simulink model "test"  (R2025b)
settings: Solver=ode8  StartTime=0.0  StopTime=4  RelTol=1e-3
libraries: simulink x4, dspfdesign x3, Monika x2
settings Model: VariantFading=off  Creator=maxim  LastModifiedBy=maxim

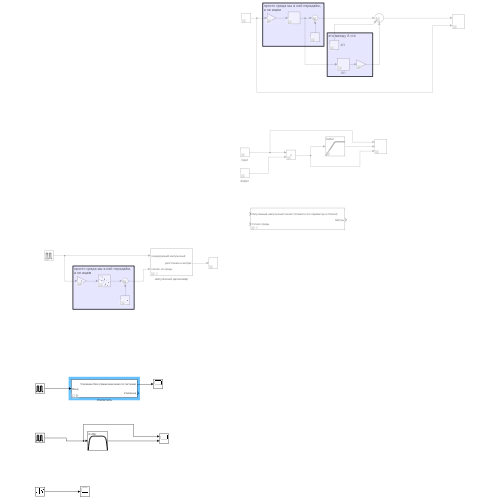
[thumbnail: Simulink's stored preview of the top-level diagram]
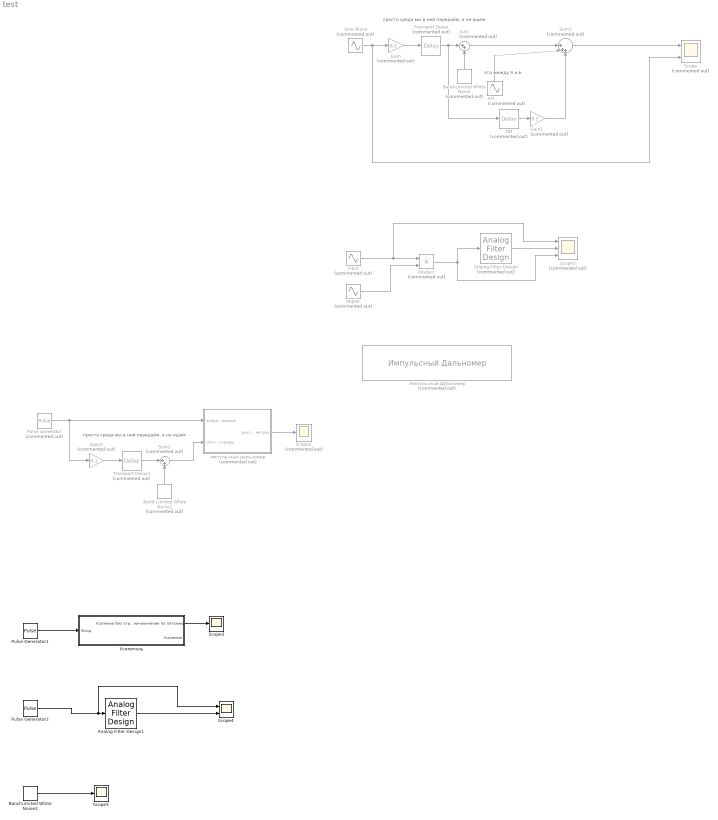
== system test ==
  note: это между А и Ь
  note: просто среда мы в ней передаём,
      | а не ищем
  note: просто среда мы в ней передаём,
      | а не ищем
  Analog Filter Design : dspfdesign/Analog Filter Design  Commented=on  method=Butterworth  filttype=Highpass  N=8  Wlo=20+8  Whi=80  Rp=2  Rs=40
  Analog Filter Design1 : dspfdesign/Analog Filter Design  method=Butterworth  filttype=Bandpass  N=2  Wlo=0.001  Whi=10  Rp=2  Rs=40
  Band-Limited White Noise : simulink/Sources/Band-Limited White Noise  Commented=on  Cov=[0.001]  Ts=0.001  seed=[23341]
  Band-Limited White Noise1 : simulink/Sources/Band-Limited White Noise  Commented=on  Cov=[0.001]  Ts=0.001  seed=[23341]
  Band-Limited White Noise2 : simulink/Sources/Band-Limited White Noise  Cov=0  Ts=0.00001  seed=[23341]
  Gain : Gain  Commented=on  Gain=0.1
  Gain1 : Gain  Commented=on  Gain=0.2
  Gain2 : Gain  Commented=on  Gain=0.1
  Product : Product  Commented=on
  Pulse Generator : DiscretePulseGenerator  Commented=on  PulseType=Time based  Period=1
  Pulse Generator1 : DiscretePulseGenerator  PulseType=Time based  Period=1  PulseWidth=10
  Pulse Generator2 : DiscretePulseGenerator  PulseType=Time based  Period=1  PulseWidth=10
  Scope : Scope  Commented=on  NumInputPorts=2
      settings: ActiveDisplayYMinimum=-12.499999674694067  ActiveDisplayYMaximum=12.499999961980945
  Scope1 : Scope  Commented=on  NumInputPorts=3
      settings: ActiveDisplayYMinimum=-1.2499999762577283  ActiveDisplayYMaximum=1.2499999284292547
  Scope2 : Scope  Commented=on
      settings: ActiveDisplayYMinimum=-206249.99999999994  ActiveDisplayYMaximum=1.85625E+6  DataLoggingVariableName=ScopeData2
  Scope3 : Scope
      settings: ActiveDisplayYMinimum=-1  ActiveDisplayYMaximum=1  DataLoggingVariableName=ScopeData3
  Scope4 : Scope  NumInputPorts=2
      settings: ActiveDisplayYMinimum=-1  ActiveDisplayYMaximum=1  DataLoggingVariableName=ScopeData4
  Scope5 : Scope
      settings: ActiveDisplayYMinimum=-1  ActiveDisplayYMaximum=1  DataLoggingVariableName=ScopeData5
  Sine Wave : Sin  Commented=on  Amplitude=10  Frequency=35  SampleTime=0
  Sum : Sum  Commented=on  Inputs=|++
  Sum1 : Sum  Commented=on  Inputs=||+++
  Sum2 : Sum  Commented=on  Inputs=|++
  Transport Delay : TransportDelay  Commented=on
  Transport Delay1 : TransportDelay  Commented=on  DelayTime=0.01
  dopler : Sin  Commented=on  Frequency=8  SampleTime=0
  input : Sin  Commented=on  Frequency=20  SampleTime=0
  АП : Sin  Commented=on  Amplitude=4  Frequency=40  SampleTime=0
  Импульсный Дальномер : Monika/Импульсный Дальномер  Commented=on  T=10  q=10
  ПП : TransportDelay  Commented=on
  Усилитель : Subsystem  AncestorBlock=Monika/Усилитель  mask(Усилитель){Gain=80, dBell_G=Децибелы, RSN=25, dBell_RSN=Децибелы, PowerLimit=10, fl=0.001, fh=10}
      mask prompts: Gain "Усиление"; dBell_G "Множитель усиления"; RSN "ОСШ"; dBell_RSN "Множитель ОСШ"; PowerLimit "Ограничение питания (В)"; fl "Нижняя частота пропускания (Гц)"; fh "Верхняя частота пропускания (Гц)"
      mask help: Блок эмитирует реальный усилитель, усиливая входной сигнал и выводя его с помехами с заданым ОСШ. Также усилитель учитывает ограничение питания сети, к которой он подключён.
      mask Help: Как вы сломали усилитель??? Напишите нам на  Github: https://github.com/Maximon0101/Monika_SimulinkLib
  импульсный дальномер : Subsystem  Commented=on  mask{T_clc=0.000228}
      mask prompts: T_clc "период тактирующего сигнала"
  wires:
  Gain/1 -> Transport Delay/1
  Sine Wave/1 -> Scope/2, Gain/1
  Band-Limited White Noise/1 -> Sum/2
  Transport Delay/1 -> ПП/1, Sum/1
  Sum/1 -> Sum1/1
  АП/1 -> Sum1/2
  ПП/1 -> Gain1/1
  Gain1/1 -> Sum1/3
  Sum1/1 -> Scope/1
  dopler/1 -> Product/2
  input/1 -> Scope1/1, Product/1
  Product/1 -> Analog Filter Design/1, Scope1/3
  Analog Filter Design/1 -> Scope1/2
  Band-Limited White Noise1/1 -> Sum2/2
  Transport Delay1/1 -> Sum2/1
  Gain2/1 -> Transport Delay1/1
  Pulse Generator/1 -> импульсный дальномер/1(зондирующий импульсный), Gain2/1
  Sum2/1 -> импульсный дальномер/2(сигнал из среды)
  импульсный дальномер/1(расстояние в метрах) -> Scope2/1
  Pulse Generator1/1 -> Усилитель/1(Вход)
  Усилитель/1(Усиление без ограниченичения по питанию) -> Scope3/1
  Analog Filter Design1/1 -> Scope4/2
  Pulse Generator2/1 -> Scope4/1, Analog Filter Design1/1
  Band-Limited White Noise2/1 -> Scope5/1

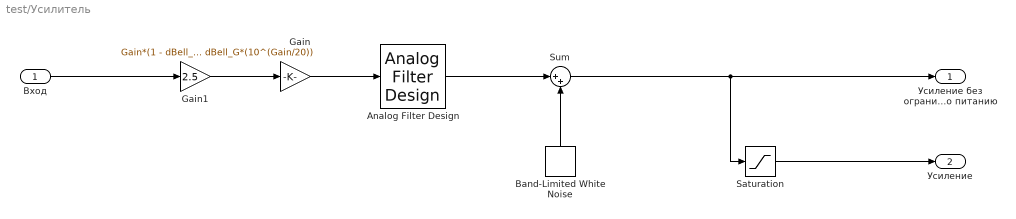
== system test/Усилитель ==
  Вход : Inport
  Analog Filter Design : dspfdesign/Analog Filter Design  method=Butterworth  filttype=Bandpass  N=2  Wlo=fl  Whi=fh  Rp=2  Rs=40
  Band-Limited White Noise : simulink/Sources/Band-Limited White Noise  Cov=( 1*(1 - dBell_G) + dBell_G*(10^(1/20)) )/ ( RSN*(1 - dBell_RSN) + dBell_RSN*(10^(RSN/20)) )  Ts=0.00001  seed=[23341]
  Gain : Gain  Gain=Gain*(1 - dBell_G) + dBell_G*(10^(Gain/20))
  Gain1 : Gain  Gain=2.5
  Saturation : Saturate  UpperLimit=PowerLimit  LowerLimit=-PowerLimit
  Sum : Sum  Inputs=|++
  Усиление без ограниченичения по питанию : Outport
  Усиление : Outport  Port=2
  wires:
  Вход/1 -> Gain1/1
  Band-Limited White Noise/1 -> Sum/2
  Saturation/1 -> Усиление/1
  Gain1/1 -> Gain/1
  Gain/1 -> Analog Filter Design/1
  Analog Filter Design/1 -> Sum/1
  Sum/1 -> Saturation/1, Усиление без ограниченичения по питанию/1

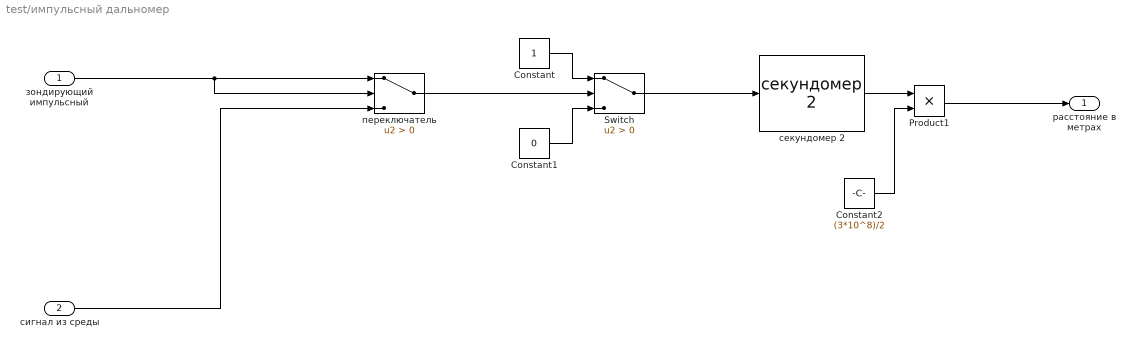
== system test/импульсный дальномер ==
  зондирующий импульсный : Inport
  сигнал из среды : Inport  Port=2
  Constant : Constant
  Constant1 : Constant  Value=0
  Constant2 : Constant  Value=(3*10^8)/2
  Product1 : Product
  Switch : Switch  Criteria=u2 > Threshold  SaturateOnIntegerOverflow=off  InputSameDT=off
  переключатель : Switch  Criteria=u2 > Threshold  SaturateOnIntegerOverflow=off  InputSameDT=off
  секундомер 2 : Monika/секундомер 2  T_clk=T_clc
  расстояние в метрах : Outport
  wires:
  Constant/1 -> Switch/1
  переключатель/1 -> Switch/2
  зондирующий импульсный/1 -> переключатель/2, переключатель/1
  Constant1/1 -> Switch/3
  Constant2/1 -> Product1/2
  Switch/1 -> секундомер 2/1
  секундомер 2/1 -> Product1/1
  Product1/1 -> расстояние в метрах/1
  сигнал из среды/1 -> переключатель/3
